simulink model "friction"  (R2018b)
settings: Solver=VariableStepAuto  StartTime=0.0  StopTime=10.0  RelTol=1e-3
settings Model: Creator=lpa1  LastModifiedBy=lpa1

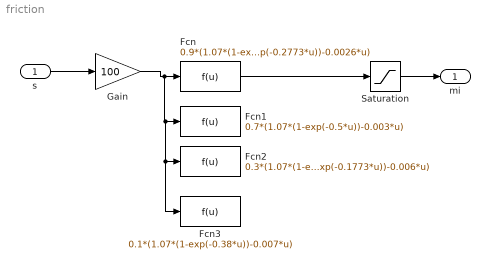
== system friction ==
  "s " : Inport
  Fcn : Fcn  Expr=0.9*(1.07*(1-exp(-0.2773*u))-0.0026*u)
  Fcn1 : Fcn  Expr=0.7*(1.07*(1-exp(-0.5*u))-0.003*u)
  Fcn2 : Fcn  Expr=0.3*(1.07*(1-exp(-0.1773*u))-0.006*u)
  Fcn3 : Fcn  Expr=0.1*(1.07*(1-exp(-0.38*u))-0.007*u)
  Gain : Gain  Gain=100
  Saturation : Saturate  UpperLimit=1  LowerLimit=0
  mi : Outport
  wires:
  "s "/1 -> Gain/1
  Gain/1 -> Fcn3/1, Fcn2/1, Fcn1/1, Fcn/1
  Fcn/1 -> Saturation/1
  Saturation/1 -> mi/1
